simulink subsystem "set_reset_ff"  (R2020b)
settings: Solver=VariableStepAuto  StartTime=0.0  StopTime=10.0  RelTol=1e-3
values from neighbouring files (symbols this model uses):
  Ts = 1/SIM.fs    [passthru_setup.m]
settings Model: Creator=Jonpe  LastModifiedBy=brian

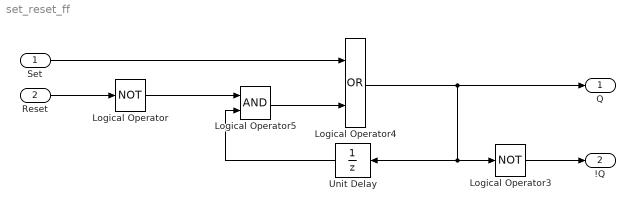
== system set_reset_ff ==
  Set : Inport  OutDataTypeStr=boolean
  Reset : Inport  Port=2  OutDataTypeStr=boolean  SampleTime=Ts
  Logical Operator : Logic  Operator=NOT  AllPortsSameDT=off  OutDataTypeStr=boolean
  Logical Operator3 : Logic  Operator=NOT  AllPortsSameDT=off  OutDataTypeStr=boolean
  Logical Operator4 : Logic  Operator=OR  AllPortsSameDT=off  OutDataTypeStr=boolean
  Logical Operator5 : Logic  AllPortsSameDT=off  OutDataTypeStr=boolean
  Unit Delay : UnitDelay  SampleTime=-1  HasFrameUpgradeWarning=on
  Q : Outport  VectorParamsAs1DForOutWhenUnconnected=off
  !Q : Outport  Port=2  VectorParamsAs1DForOutWhenUnconnected=off
  wires:
  Logical Operator5/1 -> Logical Operator4/2
  Logical Operator4/1 -> Q/1, Logical Operator3/1, Unit Delay/1
  Unit Delay/1 -> Logical Operator5/2
  Logical Operator3/1 -> !Q/1
  Set/1 -> Logical Operator4/1
  Logical Operator/1 -> Logical Operator5/1
  Reset/1 -> Logical Operator/1
